simulink model "validar_espacio_estado_sistema_planetario_simulink"  (R2017b)
settings: Solver=VariableStepAuto  StartTime=0.0  StopTime=31536000  FixedStep=4000  RelTol=1e-3
libraries: simulink x2
settings Model: Creator=xmax1  LastModifiedBy=xmax1

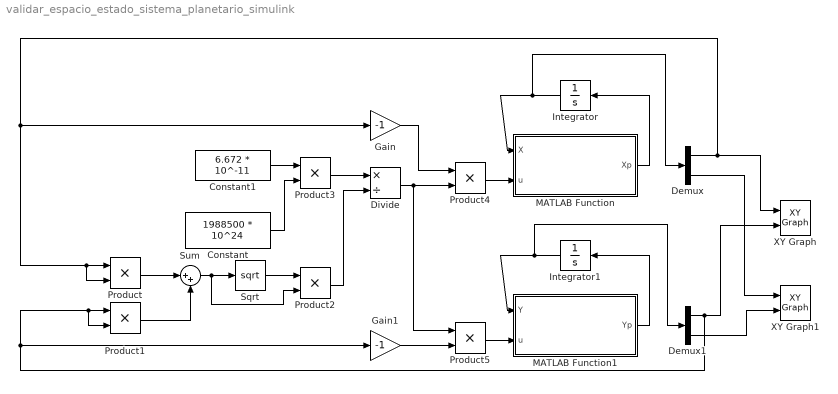
== system validar_espacio_estado_sistema_planetario_simulink ==
  Constant : Constant  Value=1988500 * 10^24
  Constant1 : Constant  Value=6.672 * 10^-11
  Demux : Demux  Outputs=2
  Demux1 : Demux  Outputs=2
  Divide : Product  Inputs=*/
  Gain : Gain  Gain=-1
  Gain1 : Gain  Gain=-1
  Integrator : Integrator  InitialCondition=[(149.6 * 1000 * 10^6)*sin(pi/4) ; -29800*sin(pi/4)]
  Integrator1 : Integrator  InitialCondition=[(149.6 * 1000 * 10^6)*sin(pi/4) ; -29800*cos(3*pi/4)]
  MATLAB Function : MATLAB Function  TreatAsAtomicUnit=on
  MATLAB Function1 : MATLAB Function  TreatAsAtomicUnit=on
  Product{,1..5} (6 alike) : Product
  Sqrt : Sqrt  SaturateOnIntegerOverflow=on
  Sum : Sum  Inputs=|++
  XY Graph : simulink/Sinks/XY Graph  xmin=-149.6 * 1000 * 10^6  xmax=149.6 * 1000 * 10^6  ymin=-149.6 * 1000 * 10^6  ymax=149.6 * 1000 * 10^6  st=-1
  XY Graph1 : simulink/Sinks/XY Graph  xmin=-30000  xmax=30000  ymin=-30000  ymax=30000  st=-1
  wires:
  MATLAB Function/1(Xp) -> Integrator/1
  Integrator/1 -> Demux/1, MATLAB Function/1(X)
  Integrator1/1 -> Demux1/1, MATLAB Function1/1(Y)
  MATLAB Function1/1(Yp) -> Integrator1/1
  Product/1 -> Sum/1
  Product1/1 -> Sum/2
  Sum/1 -> Product2/2, Sqrt/1
  Sqrt/1 -> Product2/1
  Constant1/1 -> Product3/1
  Constant/1 -> Product3/2
  Product3/1 -> Divide/1
  Product2/1 -> Divide/2
  Product4/1 -> MATLAB Function/2(u)
  Gain/1 -> Product4/1
  Divide/1 -> Product5/1, Product4/2
  Gain1/1 -> Product5/2
  Product5/1 -> MATLAB Function1/2(u)
  Demux/2 -> XY Graph1/1
  Demux1/2 -> XY Graph1/2
  Demux/1 -> Product/2, Product/1, Gain/1, XY Graph/1
  Demux1/1 -> Product1/2, Product1/1, Gain1/1, XY Graph/2

== matlab function validar_espacio_estado_sistema_planetario_simulink/MATLAB Function1 ==
  data: Y input; u input; Yp output
function Yp = sistema_planetario_y(Y, u)
A = [ 0, 1 ; 0, 0 ];
B = [ 0 ; 1 ];
Yp = A*Y + B*u;

== matlab function validar_espacio_estado_sistema_planetario_simulink/MATLAB Function ==
  data: X input; u input; Xp output
function Xp = sistema_planetario_x(X, u)
A = [ 0, 1 ; 0, 0 ];
B = [ 0 ; 1 ];
Xp = A*X + B*u;
